simulink model "FullHopper_baseline"  (R2020a)
settings: Solver=ode4  StartTime=0.0  StopTime=7.5  FixedStep=0.0005  RelTol=1e-3
model workspace (MAT data in the model file):
  T_stim = 0.4
  amplitude = 1
settings Model: OrderedModelArguments=off  Creator=jmei13  LastModifiedBy=jmei13
settings DebuggingCC: AlgebraicLoopMsg=none  ArtificialAlgebraicLoopMsg=none  UnconnectedInputMsg=none  UnconnectedOutputMsg=none  UnconnectedLineMsg=none

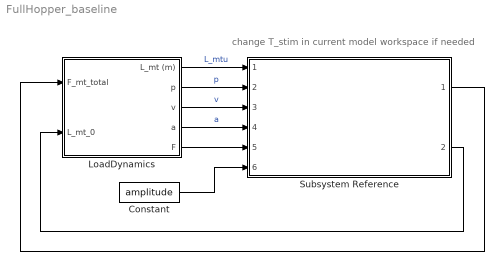
== system FullHopper_baseline ==
  note: change T_stim in current model workspace if needed
  Constant : Constant  Value=amplitude
  LoadDynamics : Subsystem
  Subsystem Reference : Subsystem  ReferencedSubsystem=muscle_dynamics_subsystem
  wires:
  LoadDynamics/1(L_mt (m)) -> Subsystem Reference/1  "L_mtu"
  LoadDynamics/2(p) -> Subsystem Reference/2  "p"
  LoadDynamics/3(v) -> Subsystem Reference/3  "v"
  LoadDynamics/4(a) -> Subsystem Reference/4  "a"
  LoadDynamics/5(F) -> Subsystem Reference/5
  Constant/1 -> Subsystem Reference/6
  Subsystem Reference/1 -> LoadDynamics/1(F_mt_total)
  Subsystem Reference/2 -> LoadDynamics/2(L_mt_0)

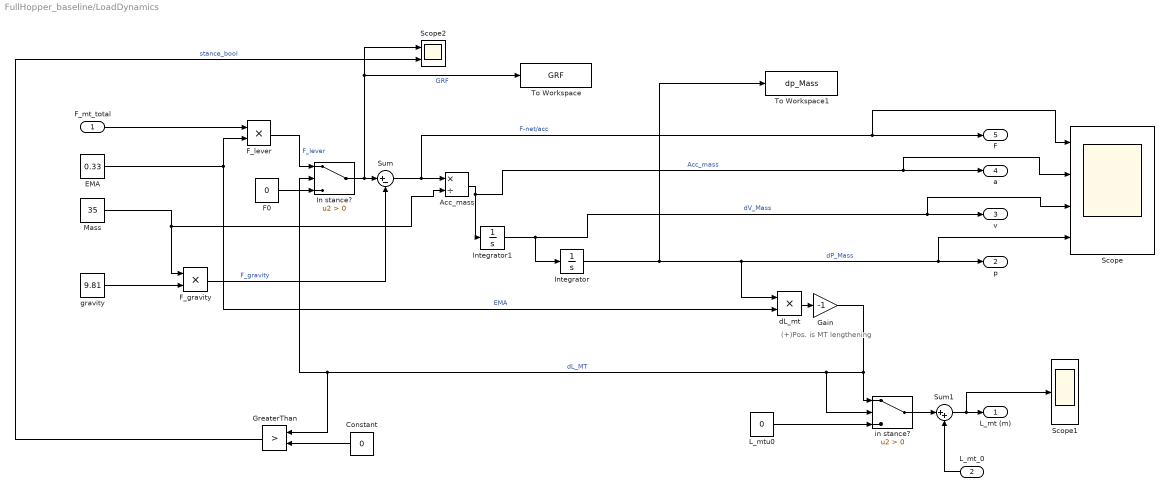
== system FullHopper_baseline/LoadDynamics ==
  note: (+)Pos. is MT
      | lengthening
  F_mt_total : Inport
  L_mt_0 : Inport  Port=2
  Acc_mass : Product  Inputs=*/
  Constant : Constant  Value=0
  EMA : Constant  Value=0.33
  F0 : Constant  Value=0
  F_gravity : Product  RndMeth=Zero
  F_lever : Product  RndMeth=Zero
  Gain : Gain  Gain=-1
  GreaterThan : RelationalOperator  Operator=>  OutDataTypeStr=boolean  RndMeth=Simplest
  In stance? : Switch  Criteria=u2 > Threshold
  Integrator : Integrator  InitialCondition=0.1
  Integrator1 : Integrator
  L_mtu0 : Constant  Value=0
  Mass : Constant  Value=35
  Scope : Scope  NumInputPorts=4
  Scope1 : Scope
  Scope2 : Scope  NumInputPorts=2
  Sum : Sum  Inputs=|+-
  Sum1 : Sum  Inputs=|++
  To Workspace : ToWorkspace  VariableName=GRF  SaveFormat=Timeseries  SampleTime=-1
  To Workspace1 : ToWorkspace  VariableName=dp_Mass  SaveFormat=Timeseries  SampleTime=-1
  dL_mt : Product  RndMeth=Zero
  gravity : Constant  Value=9.81
  "in stance? " : Switch  Criteria=u2 > Threshold
  L_mt (m) : Outport
  p : Outport  Port=2
  v : Outport  Port=3
  a : Outport  Port=4
  F : Outport  Port=5
  wires:
  Integrator1/1 -> Integrator/1, Scope/3, v/1  "dV_Mass"
  Sum1/1 -> Scope1/1, L_mt (m)/1
  L_mt_0/1 -> Sum1/2
  Acc_mass/1 -> Integrator1/1, Scope/2, a/1  "Acc_mass"
  F0/1 -> In stance?/3
  Sum/1 -> Scope/1, F/1, Acc_mass/1  "F-net/acc"
  F_mt_total/1 -> F_lever/1
  Gain/1 -> "in stance? "/2, GreaterThan/1, In stance?/2, "in stance? "/1  "dL_MT"
  dL_mt/1 -> Gain/1
  F_lever/1 -> In stance?/1  "F_lever"
  Integrator/1 -> To Workspace1/1, dL_mt/1, Scope/4, p/1  "dP_Mass"
  F_gravity/1 -> Sum/2  "F_gravity"
  EMA/1 -> F_lever/2, dL_mt/2  "EMA"
  gravity/1 -> F_gravity/2
  Mass/1 -> Acc_mass/2, F_gravity/1
  L_mtu0/1 -> "in stance? "/3
  In stance?/1 -> Scope2/1, To Workspace/1, Sum/1  "GRF"
  "in stance? "/1 -> Sum1/1
  Constant/1 -> GreaterThan/2
  GreaterThan/1 -> Scope2/2  "stance_bool"
